simulink model "Simulink_Test_Example"  (R2025b)
settings: Solver=VariableStepAuto  StartTime=0.0  StopTime=10.0  RelTol=1e-3
settings Model: Creator=georg  LastModifiedBy=P28500

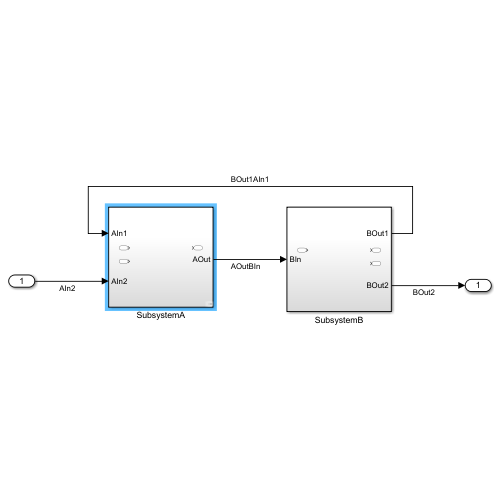
[thumbnail: Simulink's stored preview of the top-level diagram]
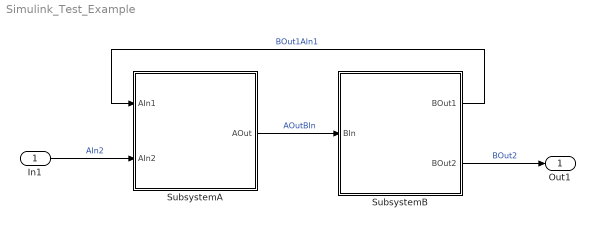
== system Simulink_Test_Example ==
  In1 : Inport
  SubsystemA : Subsystem
  SubsystemB : Subsystem
  Out1 : Outport
  wires:
  SubsystemA/1(AOut) -> SubsystemB/1(BIn)  "AOutBIn"
  SubsystemB/1(BOut1) -> SubsystemA/1(AIn1)  "BOut1AIn1"
  In1/1 -> SubsystemA/2(AIn2)  "AIn2"
  SubsystemB/2(BOut2) -> Out1/1  "BOut2"

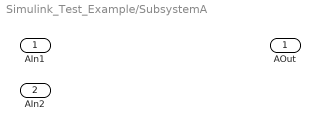
== system Simulink_Test_Example/SubsystemA ==
  AIn1 : Inport
  AIn2 : Inport  Port=2
  AOut : Outport

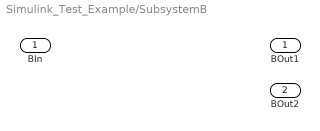
== system Simulink_Test_Example/SubsystemB ==
  BIn : Inport
  BOut1 : Outport
  BOut2 : Outport  Port=2
